simulink model "MBSE_Project_SunRoof_manual"  (R2020b)
settings: Solver=FixedStepAuto  StartTime=0.0  StopTime=90  FixedStep=10  RelTol=1e-3
undefined symbols (not defined in the file): sigbuilder_block
settings Model: Creator=99003747  LastModifiedBy=99003747

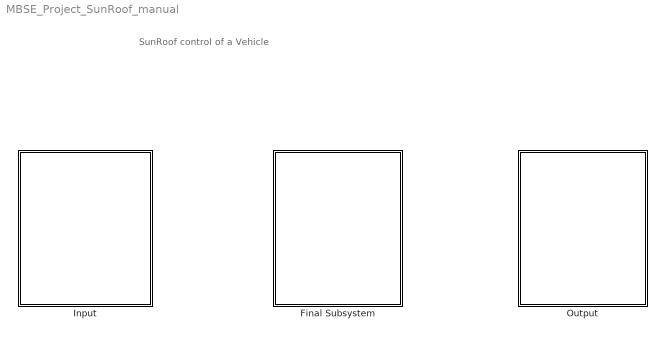
== system MBSE_Project_SunRoof_manual ==
  note: SunRoof control of a Vehicle
  Final Subsystem : Subsystem
  Input : Subsystem
  Output : Subsystem

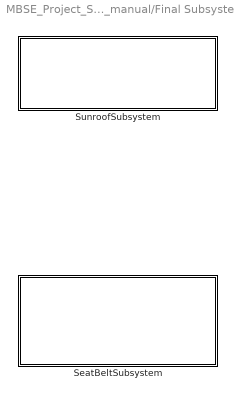
== system MBSE_Project_SunRoof_manual/Final Subsystem ==
  SeatBeltSubsystem : Subsystem
  SunroofSubsystem : Subsystem

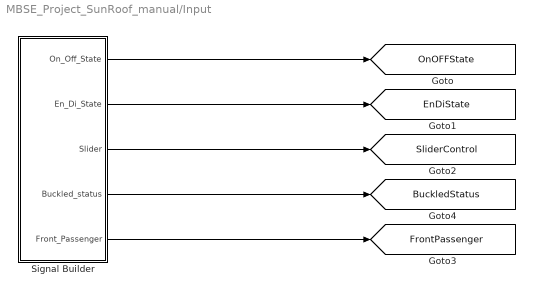
== system MBSE_Project_SunRoof_manual/Input ==
  Signal Builder : Subsystem  Tag=STV Subsys  LoadFcn=sigbuilder_block('load');  StartFcn=sigbuilder_block('start');  StopFcn=sigbuilder_block('stop');  ClipboardFcn=sigbuilder_block('clipboard');  mask(Sigbuilder block){tuvar=[0:10]}
      mask help: Simulink:masks:SigbuilderBlock_MD
      mask init:
      | if ~strcmp(get_param(bdroot(gcbh),'SimulationStatus'),'stopped') tuvar = sigbuilder_block('maskInit'); end
      settings: CopyFcn=sigbuilder_block('copy');  DeleteFcn=sigbuilder_block('delete');  ModelCloseFcn=sigbuilder_block('modelClose');  PreSaveFcn=sigbuilder_block('preSave');  PauseFcn=sigbuilder_block('pause');  ContinueFcn=sigbuilder_block('continue');  NameChangeFcn=sigbuilder_block('namechange');  OpenFcn=sigbuilder_block('open',[437.6 199.2 550.4 400 ]);  CloseFcn=sigbuilder_block('close');
      mask Display: plot(0, 0, 100, 100,[2, 2, 32, 32, 2], [68, 8, 8, 68, 68],[32, 2], [38, 38], [32, 19, 2],[53, 60, 44], [32, 17, 17, 2],[16, 16, 31, 31]);txt = getActiveGroup(gcbh);text(2, 100, txt,'verticalAlignment', 'top');
  tag scope: BuckledStatus=global, EnDiState=global, FrontPassenger=global, OnOFFState=global, SliderControl=global
  wires:
  Signal Builder/2(En_Di_State) -> [EnDiState]
  Signal Builder/3(Slider) -> [SliderControl]
  Signal Builder/4(Buckled_status) -> [BuckledStatus]
  Signal Builder/5(Front_Passenger) -> [FrontPassenger]
  Signal Builder/1(On_Off_State) -> [OnOFFState]

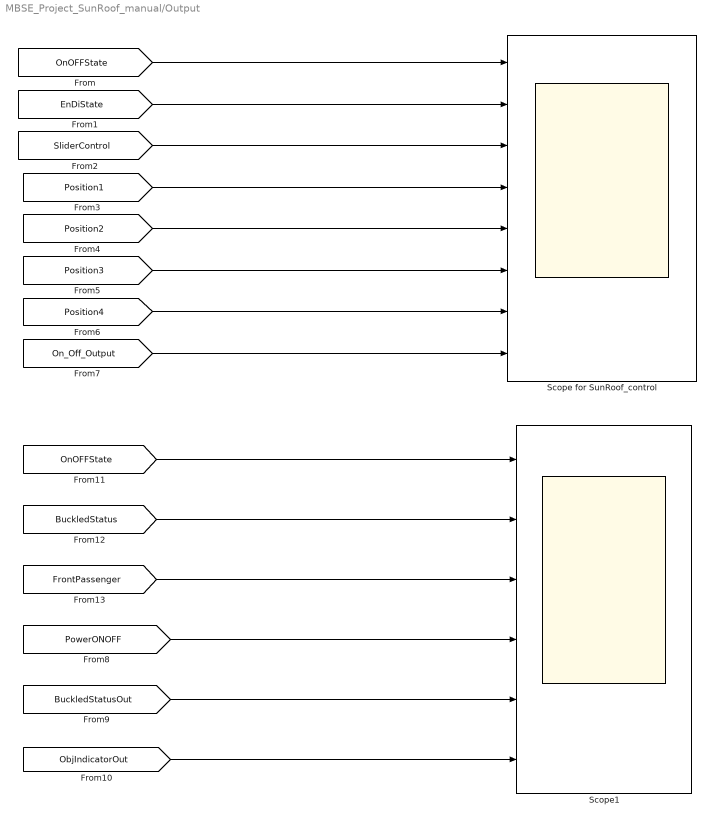
== system MBSE_Project_SunRoof_manual/Output ==
  Scope for SunRoof_control : Scope  NumInputPorts=8
  Scope1 : Scope  NumInputPorts=6
  wires:
  [OnOFFState] -> Scope for SunRoof_control/1
  [EnDiState] -> Scope for SunRoof_control/2
  [SliderControl] -> Scope for SunRoof_control/3
  [Position1] -> Scope for SunRoof_control/4
  [Position2] -> Scope for SunRoof_control/5
  [Position3] -> Scope for SunRoof_control/6
  [Position4] -> Scope for SunRoof_control/7
  [On_Off_Output] -> Scope for SunRoof_control/8
  [OnOFFState] -> Scope1/1
  [BuckledStatus] -> Scope1/2
  [FrontPassenger] -> Scope1/3
  [PowerONOFF] -> Scope1/4
  [BuckledStatusOut] -> Scope1/5
  [ObjIndicatorOut] -> Scope1/6

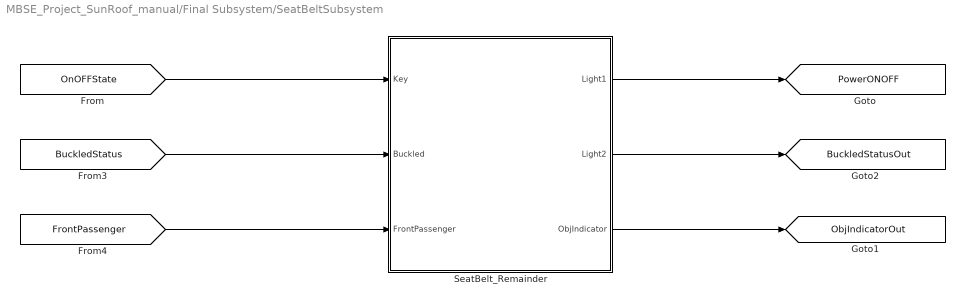
== system MBSE_Project_SunRoof_manual/Final Subsystem/SeatBeltSubsystem ==
  SeatBelt_Remainder : Stateflow chart  TreatAsAtomicUnit=on
  tag scope: BuckledStatusOut=global, ObjIndicatorOut=global, PowerONOFF=global
  wires:
  [OnOFFState] -> SeatBelt_Remainder/1(Key)
  [BuckledStatus] -> SeatBelt_Remainder/2(Buckled)
  [FrontPassenger] -> SeatBelt_Remainder/3(FrontPassenger)
  SeatBelt_Remainder/1(Light1) -> [PowerONOFF]
  SeatBelt_Remainder/2(Light2) -> [BuckledStatusOut]
  SeatBelt_Remainder/3(ObjIndicator) -> [ObjIndicatorOut]

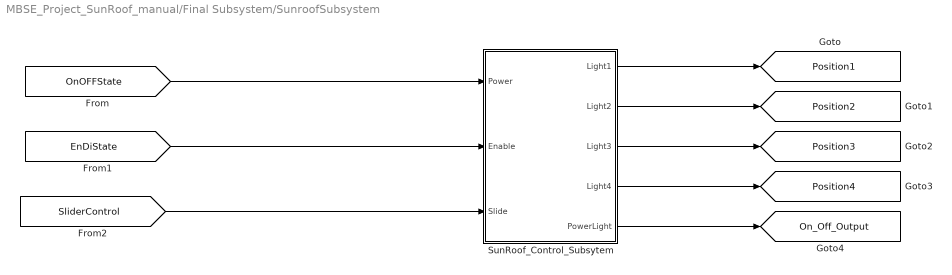
== system MBSE_Project_SunRoof_manual/Final Subsystem/SunroofSubsystem ==
  SunRoof_Control_Subsytem : Subsystem
  tag scope: On_Off_Output=global, Position1=global, Position2=global, Position3=global, Position4=global
  wires:
  [OnOFFState] -> SunRoof_Control_Subsytem/1(Power)
  SunRoof_Control_Subsytem/3(Light3) -> [Position3]
  [SliderControl] -> SunRoof_Control_Subsytem/3(Slide)
  [EnDiState] -> SunRoof_Control_Subsytem/2(Enable)
  SunRoof_Control_Subsytem/4(Light4) -> [Position4]
  SunRoof_Control_Subsytem/2(Light2) -> [Position2]
  SunRoof_Control_Subsytem/1(Light1) -> [Position1]
  SunRoof_Control_Subsytem/5(PowerLight) -> [On_Off_Output]

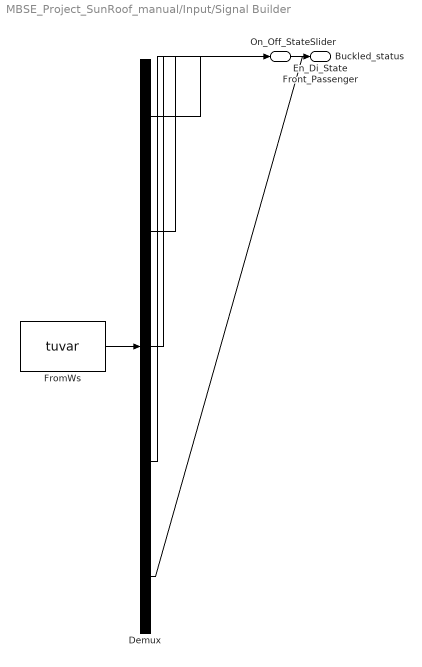
== system MBSE_Project_SunRoof_manual/Input/Signal Builder ==
  Demux : Demux  Tag=STV Demux  Outputs=5
      settings: DisplayOption=none
  FromWs : FromWorkspace  Tag=STV FromWs  VariableName=tuvar
      SigBuilderData=|
      | common.afterFinalStr = 'Extrapolate'
      | common.sampleTime = 0
      | dataSet.timeRange = [0 82]
      | dataSet.name = 'Sheet1'
      | sbobj.Name = 'Signal Builder'
      | sbobj.Groups.Name = 'Sheet1'
      | sbobj.Groups.Signals(1).Name = 'On_Off_State'
      | sbobj.Groups.Signals(1).XData = [0 6 15 22 29.5 37 44.5 52 59.5 67 74.5 82]
      | sbobj.Groups.Signals(1).YData = [0 0 0 0 1 1 1 1 1 1 1 1]
      | sbobj.Groups.Signals(2).Name = 'En_Di_State'
      | sbobj.Groups.Signals(2).XData = [0 6 15 22 29.5 37 44.5 52 59.5 67 74.5 82]
      | sbobj.Groups.Signals(2).YData = [0 0 0 0 0 0 0 0 1 1 1 1]
      | sbobj.Groups.Signals(3).Name = 'Slider'
      | sbobj.Groups.Signals(3).XData = [0 6 15 22 29.5 37 44.5 52 59.5 67 74.5 82]
      | sbobj.Groups.Signals(3).YData = [10 30 60 80 10 30 60 80 10 30 60 80]
      | sbobj.Groups.Signals(4).Name = 'Buckled_status'
      | sbobj.Groups.Signals(4).XData = [0 6 15 22 29.5 37 44.5 52 59.5 67 74.5 82]
      | sbobj.Groups.Signals(4).YData = [0 0 0 0 0 1 1 1 1 0 0 0]
      | sbobj.Groups.Signals(5).Name = 'Front_Passenger'
      | sbobj.Groups.Signals(5).XData = [0 6 15 22 29.5 37 44.5 52 59.5 67 74.5 82]
      | sbobj.Groups.Signals(5).YData = [0 0 1 1 1 1 0 0 0 0 1 1]
      | sbobj.Groups.TimeRange = [0 82]
  On_Off_State : Outport  Tag=STV Outport
  En_Di_State : Outport  Tag=STV Outport  Port=2
  Slider : Outport  Tag=STV Outport  Port=3
  Buckled_status : Outport  Tag=STV Outport  Port=4
  Front_Passenger : Outport  Tag=STV Outport  Port=5
  wires:
  Demux/1 -> On_Off_State/1
  FromWs/1 -> Demux/1
  Demux/2 -> En_Di_State/1
  Demux/3 -> Slider/1
  Demux/4 -> Buckled_status/1
  Demux/5 -> Front_Passenger/1

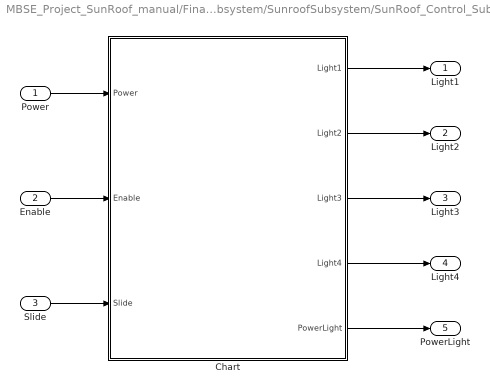
== system MBSE_Project_SunRoof_manual/Final Subsystem/SunroofSubsystem/SunRoof_Control_Subsytem ==
  Power : Inport
  Enable : Inport  Port=2
  Slide : Inport  Port=3
  Chart : Stateflow chart  TreatAsAtomicUnit=on
  Light1 : Outport
  Light2 : Outport  Port=2
  Light3 : Outport  Port=3
  Light4 : Outport  Port=4
  PowerLight : Outport  Port=5
  wires:
  Slide/1 -> Chart/3(Slide)
  Chart/3(Light3) -> Light3/1
  Chart/1(Light1) -> Light1/1
  Chart/2(Light2) -> Light2/1
  Enable/1 -> Chart/2(Enable)
  Power/1 -> Chart/1(Power)
  Chart/4(Light4) -> Light4/1
  Chart/5(PowerLight) -> PowerLight/1

== stateflow chart MBSE_Project_SunRoof_manual/Final Subsystem/SunroofSubsystem/SunRoof_Control_Subsytem/Chart ==
  state PowerOff
    entry:
    PowerLight=0;
    Light1=0;
    Light2=0;
    Light3=0;
    Light4=0;
  state PowerOn
    entry:
    PowerLight=1;
    Light1=0;
    Light2=0;
    Light3=0;
    Light4=0;
  state RoofPosition1
    entry:
    Light1=1;
    Light2=0;
    Light3=0;
    Light4=0;
  state RoofPosition2
    entry:
    Light1=1;
    Light2=1;
    Light3=0;
    Light4=0;
  state RoofPosition4
    entry:
    Light1=1;
    Light2=1;
    Light3=1;
    Light4=1;
  state RoofPosition3
    entry:
    Light1=1;
    Light2=1;
    Light3=1;
    Light4=0;
  (default) -> PowerOff
  PowerOn -> RoofPosition4 [order 2] : [Enable ==1 && Slide>75 && Slide<=100]
  PowerOff -> PowerOn : [Power == 1  ]
  RoofPosition4 -> PowerOn [order 1] : [Enable == 0]
  PowerOn -> PowerOff [order 5] : [Power == 0]
  RoofPosition1 -> PowerOn [order 4] : [Enable ==1 && Slide<=0 && Slide>25]
  PowerOn -> RoofPosition1 [order 4] : [Enable ==1 && Slide>0 && Slide<25]
  RoofPosition1 -> PowerOff [order 2] : [Power == 0]
  RoofPosition1 -> PowerOn [order 1] : [Enable == 0]
  RoofPosition4 -> PowerOff [order 2] : [Power == 0]
  PowerOn -> RoofPosition2 [order 3] : [Enable ==1 && Slide>=25 && Slide<50]
  RoofPosition2 -> PowerOn [order 1] : [Enable == 0]
  RoofPosition3 -> PowerOn [order 1] : [Enable == 0]
  PowerOn -> RoofPosition3 [order 1] : [Enable ==1 && Slide>=50 && Slide<75]
  RoofPosition2 -> PowerOff [order 2] : [Power == 0]
  RoofPosition3 -> PowerOff [order 2] : [Power == 0]
  RoofPosition2 -> RoofPosition1 [order 3] : [Enable ==1 && Slide<=25 && Slide>0]
  RoofPosition3 -> RoofPosition2 [order 3] : [Enable ==1 && Slide<=50 && Slide>25]
  RoofPosition4 -> RoofPosition3 [order 3] : [Enable ==1 && Slide<=75 && Slide>50]
  RoofPosition1 -> RoofPosition2 [order 3] : [Enable ==1 && Slide>=25 && Slide<50]
  RoofPosition2 -> RoofPosition3 [order 4] : [Enable ==1 && Slide>=50 && Slide<75]
  RoofPosition3 -> RoofPosition4 [order 4] : [Enable ==1 && Slide>=75 && Slide<100]
  data: Power input; Light1 output; Enable input; Light2 output; Light3 output; Light4 output; Slide input; PowerLight output

== stateflow chart MBSE_Project_SunRoof_manual/Final Subsystem/SeatBeltSubsystem/SeatBelt_Remainder ==
  state Indicator
    entry:
    ObjIndicator=1;
    state VehicleOn
      entry:
      Light1=1;
      Light2=1;
    state Chime
      entry:
      Light2=0;
    (default) -> VehicleOn
    Chime -> VehicleOn : [Light2==0]
    VehicleOn -> Chime : [Light2==1]
  state VehicleOff
    entry:
    Light1=0;
    Light2=0;
  state SeatBeltBuckled
    entry:
    Light2=0;
  state frontPassenger
    entry:
    ObjIndicator=0;
  (default) -> VehicleOff
  Indicator -> SeatBeltBuckled [order 1] : [Buckled==1]
  Indicator -> VehicleOff [order 3] : [Key==0]
  SeatBeltBuckled -> Indicator [order 1] : [Buckled==0]
  VehicleOff -> Indicator : [Key==1 ]
  SeatBeltBuckled -> VehicleOff [order 2] : [Key==0]
  frontPassenger -> SeatBeltBuckled [order 2] : [Buckled == 1]
  SeatBeltBuckled -> frontPassenger [order 3] : [Buckled == 0]
  frontPassenger -> Indicator [order 1] : [Key == 1 && FrontPassenger ==1 ]
  Indicator -> frontPassenger [order 2] : [ FrontPassenger ==0]
  frontPassenger -> VehicleOff [order 3] : [Key == 0]
  data: Light1 output; Light2 output; Key input =0; Buckled input; ObjIndicator output; FrontPassenger input
